simulink model "Task6_servo_controller"  (R2023b)
settings: Solver=VariableStepAuto  StartTime=0.0  StopTime=25  RelTol=1e-3
values from neighbouring files (symbols this model uses):
  A = [-1.7  -0.25  0; 23  -30  20; 0  -250  -720]    [A.mat]
  B = [3  0; -103  0; 0  -790]    [B.mat]
  C = [0  1  0; 0  0  1]    [C.mat]
  K1 = K(:,1:3)    [Task5_servo_control.m]    (also in Task6_servo_control.m)
  K2 = K(:,4:5)    [Task5_servo_control.m]    (also in Task6_servo_control.m)
  W = [6,0,0;0,7,0;0,0,12]    [Task6_servo_control.m]
  X0 = [1;100;200]    [Task6_servo_control.m]
  X_SP = [5;250;300]    [Task6_servo_control.m]
settings Model: Creator=25039  LastModifiedBy=25039

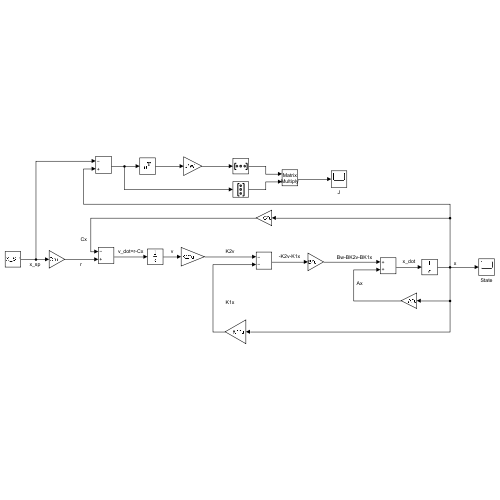
[thumbnail: Simulink's stored preview of the top-level diagram]
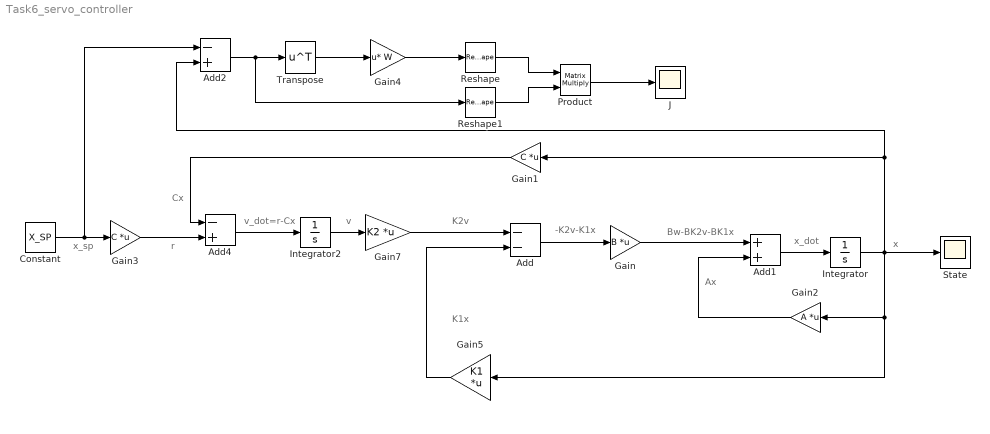
== system Task6_servo_controller ==
  note: r
  note: K2v
  note: K1x
  note: v
  note: v_dot=r-Cx
  note: Cx
  note: x
  note: x_dot
  note: Ax
  note: Bw-BK2v-BK1x
  note: -K2v-K1x
  note: x_sp
  Add : Sum  Inputs=--
  Add1 : Sum
  Add2 : Sum  Inputs=-+
  Add4 : Sum  Inputs=-+
  Constant : Constant  Value=X_SP
  Gain : Gain  Gain=B  Multiplication=Matrix(K*u)
  Gain1 : Gain  Gain=C  Multiplication=Matrix(K*u)
  Gain2 : Gain  Gain=A  Multiplication=Matrix(K*u)
  Gain3 : Gain  Gain=C  Multiplication=Matrix(K*u)
  Gain4 : Gain  Gain=W  Multiplication=Matrix(u*K)
  Gain5 : Gain  Gain=K1  Multiplication=Matrix(K*u)
  Gain7 : Gain  Gain=K2  Multiplication=Matrix(K*u)
  Integrator : Integrator  InitialCondition=X0
  Integrator2 : Integrator  InitialCondition=[0;0]
  J : Scope
  Product : Product  Multiplication=Matrix(*)
  Reshape : Reshape  OutputDimensionality=Row vector (2-D)  OutputDimensions=[1,3]
  Reshape1 : Reshape  OutputDimensionality=Column vector (2-D)  OutputDimensions=[3,1]
  State : Scope
  Transpose : Math  Operator=transpose
  wires:
  Add/1 -> Gain/1
  Gain/1 -> Add1/1
  Add1/1 -> Integrator/1
  Integrator/1 -> Add2/2, Gain1/1, State/1, Gain5/1, Gain2/1
  Gain2/1 -> Add1/2
  Add4/1 -> Integrator2/1
  Integrator2/1 -> Gain7/1
  Gain7/1 -> Add/1
  Gain5/1 -> Add/2
  Gain1/1 -> Add4/1
  Gain3/1 -> Add4/2
  Add2/1 -> Reshape1/1, Transpose/1
  Transpose/1 -> Gain4/1
  Gain4/1 -> Reshape/1
  Product/1 -> J/1
  Reshape/1 -> Product/1
  Reshape1/1 -> Product/2
  Constant/1 -> Add2/1, Gain3/1
